simulink model "FCS"  (Simulink 9.1)
settings: Solver=VariableStepAuto  StartTime=0.0  StopTime=10.0  RelTol=1e-3
values from neighbouring files (symbols this model uses):
  Controller =     [data_set.mat]
  Estimator =     [data_set.mat]
  g = 9.81    [data_set.mat]
  init =     [data_set.mat]
  Sensors =     [data_set.mat]
  Ts = 0.005    [data_set.mat]
  Vehicle =     [data_set.mat]
undefined symbols (not defined in the file or in its folder): DiscIntNeverNeededParam, Discrete, Time
libraries: F_Line_block x503, simulink x33, ctrlSharedLib x3, sharedtransform x3, sharedutil x1
(part 2 of 3)

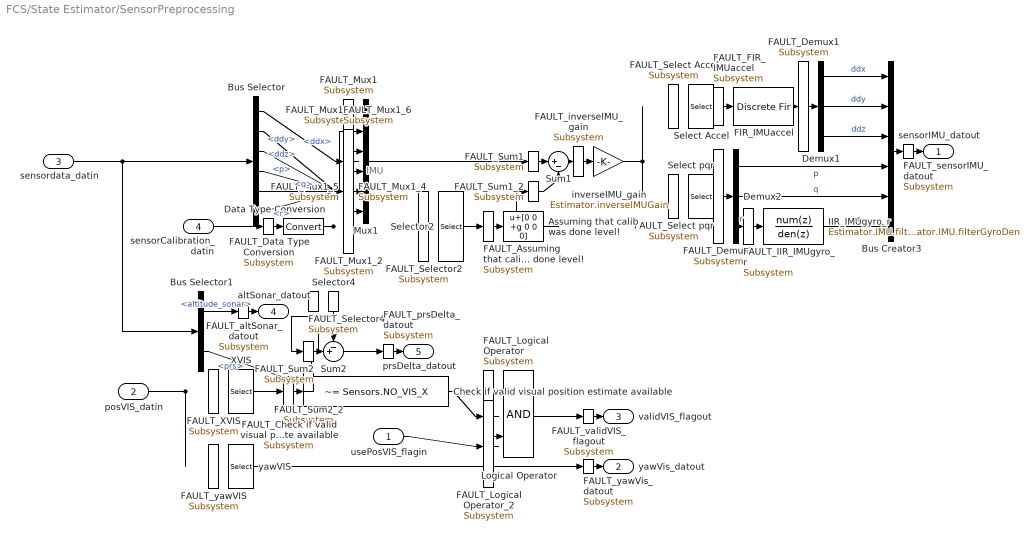
== system FCS/State Estimator/SensorPreprocessing ==
  note: IMU
  usePosVIS_flagin : Inport
  posVIS_datin : Inport  Port=2
  sensordata_datin : Inport  Port=3
  sensorCalibration_datin : Inport  Port=4
  Assuming that calib was done level! : Bias  Bias=[0 0 +g 0 0 0]
  FAULT_Assuming that calib was done level! : F_Line_block/Subsystem
  Bus Creator3 : BusCreator  Inputs=6
  Bus Selector : BusSelector  OutputSignals=ddx,ddy,ddz,p,q,r
  Bus Selector1 : BusSelector  OutputSignals=altitude_sonar,prs
  Check if valid visual position estimate available : simulink/Logic and Bit Operations/Compare To Constant  relop=~=  const=Sensors.NO_VIS_X  OutDataTypeStr=boolean
  FAULT_Check if valid visual position estimate available : F_Line_block/Subsystem
  Data Type Conversion : DataTypeConversion
  FAULT_Data Type Conversion : F_Line_block/Subsystem
  Demux1 : Demux  Outputs=3
  FAULT_Demux1 : F_Line_block/Subsystem
  Demux2 : Demux  Outputs=3
  FAULT_Demux2 : F_Line_block/Subsystem
  FIR_IMUaccel : DiscreteFir  Coefficients=Estimator.IMU.filterAccel.Coefficients
  FAULT_FIR_IMUaccel : F_Line_block/Subsystem
  IIR_IMUgyro_r : DiscreteFilter  Numerator=Estimator.IMU.filterGyroNum  Denominator=Estimator.IMU.filterGyroDen
  FAULT_IIR_IMUgyro_r : F_Line_block/Subsystem
  Logical Operator : Logic  AllPortsSameDT=off  OutDataTypeStr=boolean
  FAULT_Logical Operator : F_Line_block/Subsystem
  FAULT_Logical Operator_2 : F_Line_block/Subsystem
  Mux1 : Mux  Inputs=6
  FAULT_Mux1 : F_Line_block/Subsystem
  FAULT_Mux1_{2..6} (5 alike) : F_Line_block/Subsystem
  Select Accel : Selector  InputPortWidth=6  IndexOptions=Index vector (dialog)  Indices=[1 2 3]  OutputSizes=1
  FAULT_Select Accel : F_Line_block/Subsystem
  Select pqr : Selector  InputPortWidth=6  IndexOptions=Index vector (dialog)  Indices=[4 5 6]  OutputSizes=1
  FAULT_Select pqr : F_Line_block/Subsystem
  Selector2 : Selector  InputPortWidth=8  IndexOptions=Index vector (dialog)  Indices=[1:6]  OutputSizes=1
  FAULT_Selector2 : F_Line_block/Subsystem
  Selector4 : Selector  InputPortWidth=8  IndexOptions=Index vector (dialog)  Indices=[7]  OutputSizes=1
  FAULT_Selector4 : F_Line_block/Subsystem
  Sum1 : Sum  Inputs=|+-
  FAULT_Sum1 : F_Line_block/Subsystem
  FAULT_Sum1_2 : F_Line_block/Subsystem
  Sum2 : Sum  Inputs=-+|
  FAULT_Sum2 : F_Line_block/Subsystem
  FAULT_Sum2_2 : F_Line_block/Subsystem
  XVIS : Selector  InputPortWidth=4  IndexOptions=Index vector (dialog)  Indices=1  OutputSizes=1
  FAULT_XVIS : F_Line_block/Subsystem
  inverseIMU_gain : Gain  Gain=Estimator.inverseIMUGain  ParamDataTypeStr=single  OutDataTypeStr=single
  FAULT_inverseIMU_gain : F_Line_block/Subsystem
  yawVIS : Selector  InputPortWidth=4  IndexOptions=Index vector (dialog)  Indices=4  OutputSizes=1
  FAULT_yawVIS : F_Line_block/Subsystem
  sensorIMU_datout : Outport
  FAULT_sensorIMU_datout : F_Line_block/Subsystem
  yawVis_datout : Outport  Port=2
  FAULT_yawVis_datout : F_Line_block/Subsystem
  validVIS_flagout : Outport  Port=3
  FAULT_validVIS_flagout : F_Line_block/Subsystem
  altSonar_datout : Outport  Port=4
  FAULT_altSonar_datout : F_Line_block/Subsystem
  prsDelta_datout : Outport  Port=5
  FAULT_prsDelta_datout : F_Line_block/Subsystem
  wires:
  Select pqr/1 -> FAULT_Demux2/1
  ?FAULT_dxy_estimout_		DstPort			1/1 -> ?dxy_estimout/dstport			1
  ?FAULT_KalmanFilter_posxy/1 -> ?KalmanFilter_posxy/1
  FAULT_Demux2/1 -> Demux2/1
  Assuming that calib was done level!/1 -> FAULT_Sum1_2/1
  FAULT_Sum1_2/1 -> Sum1/2
  usePosVIS_flagin/1 -> FAULT_Logical Operator_2/1
  FAULT_Logical Operator_2/1 -> Logical Operator/2
  Check if valid visual position estimate available/1 -> FAULT_Logical Operator/1
  FAULT_Logical Operator/1 -> Logical Operator/1
  Logical Operator/1 -> FAULT_validVIS_flagout/1
  FAULT_validVIS_flagout/1 -> validVIS_flagout/1
  yawVIS/1 -> FAULT_yawVis_datout/1
  FAULT_yawVis_datout/1 -> yawVis_datout/1
  XVIS/1 -> FAULT_Check if valid visual position estimate available/1
  FAULT_Check if valid visual position estimate available/1 -> Check if valid visual position estimate available/1
  Mux1/1 -> FAULT_Sum1/1
  FAULT_Sum1/1 -> Sum1/1
  Sum2/1 -> FAULT_prsDelta_datout/1
  FAULT_prsDelta_datout/1 -> prsDelta_datout/1
  Bus Selector1/2 -> FAULT_Sum2_2/1  "<prs>"
  FAULT_Sum2_2/1 -> Sum2/2
  Selector4/1 -> FAULT_Sum2/1
  FAULT_Sum2/1 -> Sum2/1
  Bus Selector1/1 -> FAULT_altSonar_datout/1  "<altitude_sonar>"
  FAULT_altSonar_datout/1 -> altSonar_datout/1
  sensordata_datin/1 -> Bus Selector1/1, Bus Selector/1
  Bus Selector/6 -> FAULT_Mux1_6/1  "<r>"
  ?FAULT_dxy_estimout_		DstPort			1/1 -> ?dxy_estimout/dstport			1
  ?FAULT_KalmanFilter_posxy/1 -> ?KalmanFilter_posxy/1
  FAULT_Mux1_6/1 -> Mux1/6
  Bus Selector/5 -> FAULT_Mux1_5/1  "<q>"
  FAULT_Mux1_5/1 -> Mux1/5
  Bus Selector/4 -> FAULT_Mux1_4/1  "<p>"
  FAULT_Mux1_4/1 -> Mux1/4
  Bus Selector/3 -> FAULT_Mux1_3/1  "<ddz>"
  FAULT_Mux1_3/1 -> Mux1/3
  Bus Selector/2 -> FAULT_Mux1_2/1  "<ddy>"
  FAULT_Mux1_2/1 -> Mux1/2
  Bus Selector/1 -> FAULT_Mux1/1  "<ddx>"
  FAULT_Mux1/1 -> Mux1/1
  sensorCalibration_datin/1 -> FAULT_Data Type Conversion/1
  FAULT_Data Type Conversion/1 -> Data Type Conversion/1
  IIR_IMUgyro_r/1 -> Bus Creator3/6  "r"
  Demux2/3 -> FAULT_IIR_IMUgyro_r/1  "r"
  FAULT_IIR_IMUgyro_r/1 -> IIR_IMUgyro_r/1
  FIR_IMUaccel/1 -> FAULT_Demux1/1
  FAULT_Demux1/1 -> Demux1/1
  Select Accel/1 -> FAULT_FIR_IMUaccel/1
  FAULT_FIR_IMUaccel/1 -> FIR_IMUaccel/1
  inverseIMU_gain/1 -> ?FAULT_Select Accel_		DstPort			1/1, ?FAULT_Select pqr_		DstPort			1/1
  ?FAULT_Select Accel_		DstPort			1/1 -> Select Accel/dstport			1
  ?FAULT_Select pqr_		DstPort			1/1 -> Select pqr/dstport			1
  Demux2/2 -> Bus Creator3/5  "q"
  Demux2/1 -> Bus Creator3/4  "p"
  Selector2/1 -> FAULT_Assuming that calib was done level!/1
  FAULT_Assuming that calib was done level!/1 -> Assuming that calib was done level!/1
  Sum1/1 -> FAULT_inverseIMU_gain/1
  FAULT_inverseIMU_gain/1 -> inverseIMU_gain/1
  Demux1/3 -> Bus Creator3/3  "ddz"
  Demux1/2 -> Bus Creator3/2  "ddy"
  Demux1/1 -> Bus Creator3/1  "ddx"
  Bus Creator3/1 -> FAULT_sensorIMU_datout/1
  FAULT_sensorIMU_datout/1 -> sensorIMU_datout/1
  posVIS_datin/1 -> ?FAULT_XVIS_		DstPort			1/1, ?FAULT_yawVIS_		DstPort			1/1
  ?FAULT_XVIS_		DstPort			1/1 -> XVIS/dstport			1
  ?FAULT_yawVIS_		DstPort			1/1 -> yawVIS/dstport			1
  Data Type Conversion/1 -> ?FAULT_Selector2_		DstPort			1/1, ?FAULT_Selector4_		DstPort			1/1
  ?FAULT_Selector2_		DstPort			1/1 -> Selector2/dstport			1
  ?FAULT_Selector4_		DstPort			1/1 -> Selector4/dstport			1

== system FCS/controller/Attitude ==
  note: ATTITUDE
  refAttitude : Inport
  states_estim : Inport  Port=2
  Add : Sum  Inputs=+-
  FAULT_Add : F_Line_block/Subsystem
  FAULT_Add_2 : F_Line_block/Subsystem
  Bus Selector3 : BusSelector  OutputSignals=pitch,roll
  Bus Selector4 : BusSelector  OutputSignals=q,p
  D_pr : Gain  Gain=[0.002;0.003]
  FAULT_D_pr : F_Line_block/Subsystem
  Delay : Delay  DelayLength=1  InitialCondition=0
  FAULT_Delay : F_Line_block/Subsystem
  Demux : Demux  Outputs=2
  FAULT_Demux : F_Line_block/Subsystem
  Discrete-Time Integrator : DiscreteIntegrator  SampleTime=Ts  LimitOutput=on  UpperSaturationLimit=2  LowerSaturationLimit=-2  ICPrevOutput=DiscIntNeverNeededParam  ICPrevScaledInput=DiscIntNeverNeededParam
  FAULT_Discrete-Time Integrator : F_Line_block/Subsystem
  I_pr : Gain  Gain=0.01
  FAULT_I_pr : F_Line_block/Subsystem
  Mux : Mux  Inputs=2
  FAULT_Mux : F_Line_block/Subsystem
  FAULT_Mux_2 : F_Line_block/Subsystem
  Mux1 : Mux  Inputs=2
  FAULT_Mux1 : F_Line_block/Subsystem
  FAULT_Mux1_2 : F_Line_block/Subsystem
  P_pr : Gain  Gain=[0.013;0.02]
  FAULT_P_pr : F_Line_block/Subsystem
  Sum16 : Sum  Inputs=++-  AccumDataTypeStr=single  OutDataTypeStr=single  SaturateOnIntegerOverflow=on
  FAULT_Sum16 : F_Line_block/Subsystem
  FAULT_Sum16_2 : F_Line_block/Subsystem
  FAULT_Sum16_3 : F_Line_block/Subsystem
  Sum19 : Sum  Inputs=+-|
  FAULT_Sum19 : F_Line_block/Subsystem
  FAULT_Sum19_2 : F_Line_block/Subsystem
  antiWU_Gain : Gain  Gain=0.001
  FAULT_antiWU_Gain : F_Line_block/Subsystem
  tau_pitch : Outport
  FAULT_tau_pitch : F_Line_block/Subsystem
  tau_roll : Outport  Port=2
  FAULT_tau_roll : F_Line_block/Subsystem
  wires:
  Sum16/1 -> FAULT_Demux/1  "P_pr"
  FAULT_Demux/1 -> Demux/1
  antiWU_Gain/1 -> FAULT_Add_2/1
  FAULT_Add_2/1 -> Add/2
  Add/1 -> FAULT_Discrete-Time Integrator/1
  FAULT_Discrete-Time Integrator/1 -> Discrete-Time Integrator/1
  Bus Selector3/1 -> FAULT_Mux/1  "<pitch>"
  FAULT_Mux/1 -> Mux/1
  Bus Selector4/1 -> FAULT_Mux1/1  "<q>"
  FAULT_Mux1/1 -> Mux1/1
  P_pr/1 -> FAULT_Sum16/1
  FAULT_Sum16/1 -> Sum16/1
  I_pr/1 -> FAULT_Sum16_2/1
  FAULT_Sum16_2/1 -> Sum16/2
  Sum19/1 -> ?FAULT_Add_		DstPort			1/1, ?FAULT_P_pr_		DstPort			1/1  "pitch/roll error"
  ?FAULT_Add_		DstPort			1/1 -> Add/dstport			1
  ?FAULT_P_pr_		DstPort			1/1 -> P_pr/dstport			1
  Discrete-Time Integrator/1 -> ?FAULT_Delay_		DstPort			1/1, ?FAULT_I_pr_		DstPort			1/1
  ?FAULT_Delay_		DstPort			1/1 -> Delay/dstport			1
  ?FAULT_I_pr_		DstPort			1/1 -> I_pr/dstport			1
  Delay/1 -> FAULT_antiWU_Gain/1
  FAULT_antiWU_Gain/1 -> antiWU_Gain/1
  Demux/1 -> FAULT_tau_pitch/1  "tau_pitch"
  FAULT_tau_pitch/1 -> tau_pitch/1
  Demux/2 -> FAULT_tau_roll/1
  FAULT_tau_roll/1 -> tau_roll/1
  D_pr/1 -> FAULT_Sum16_3/1
  FAULT_Sum16_3/1 -> Sum16/3
  states_estim/1 -> Bus Selector3/1, Bus Selector4/1
  refAttitude/1 -> FAULT_Sum19/1
  ?FAULT_Delay_		DstPort			1/1 -> Delay/dstport			1
  ?FAULT_I_pr_		DstPort			1/1 -> I_pr/dstport			1
  FAULT_Sum19/1 -> Sum19/1
  Mux/1 -> FAULT_Sum19_2/1
  FAULT_Sum19_2/1 -> Sum19/2
  Bus Selector3/2 -> FAULT_Mux_2/1  "<roll>"
  FAULT_Mux_2/1 -> Mux/2
  Mux1/1 -> FAULT_D_pr/1
  FAULT_D_pr/1 -> D_pr/1
  Bus Selector4/2 -> FAULT_Mux1_2/1  "<p>"
  FAULT_Mux1_2/1 -> Mux1/2

== system FCS/controller/ControlMixer ==
  tau_pitch : Inport
  tau_roll : Inport  Port=2
  tau_yaw : Inport  Port=3
  totalThrust : Inport  Port=4
  Mux2 : Mux
  FAULT_Mux2 : F_Line_block/Subsystem
  FAULT_Mux2_2 : F_Line_block/Subsystem
  FAULT_Mux2_3 : F_Line_block/Subsystem
  FAULT_Mux2_4 : F_Line_block/Subsystem
  Product : Product  Multiplication=Matrix(*)  RndMeth=Zero
  FAULT_Product : F_Line_block/Subsystem
  FAULT_Product_2 : F_Line_block/Subsystem
  TorqueTotalThrustToThrustPerMotor : Constant  Value=Controller.Q2Ts  OutDataTypeStr=single
  thrusts_refout : Outport
  FAULT_thrusts_refout : F_Line_block/Subsystem
  wires:
  Product/1 -> FAULT_thrusts_refout/1
  FAULT_thrusts_refout/1 -> thrusts_refout/1
  tau_roll/1 -> FAULT_Mux2_4/1
  FAULT_Mux2_4/1 -> Mux2/4
  tau_pitch/1 -> FAULT_Mux2_3/1
  FAULT_Mux2_3/1 -> Mux2/3
  tau_yaw/1 -> FAULT_Mux2_2/1
  FAULT_Mux2_2/1 -> Mux2/2
  totalThrust/1 -> FAULT_Mux2/1
  FAULT_Mux2/1 -> Mux2/1
  TorqueTotalThrustToThrustPerMotor/1 -> FAULT_Product/1
  FAULT_Product/1 -> Product/1
  Mux2/1 -> FAULT_Product_2/1
  FAULT_Product_2/1 -> Product/2

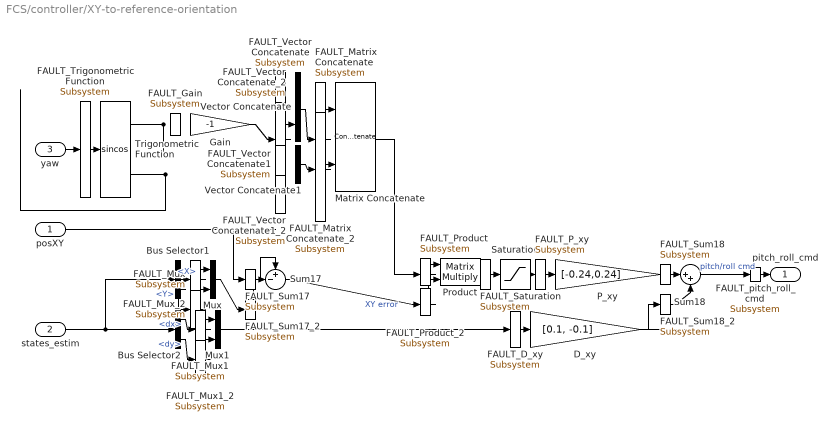
== system FCS/controller/XY-to-reference-orientation ==
  posXY : Inport
  states_estim : Inport  Port=2
  yaw : Inport  Port=3
  Bus Selector1 : BusSelector  OutputSignals=X,Y
  Bus Selector2 : BusSelector  OutputSignals=dx,dy
  D_xy : Gain  Gain=[0.1, -0.1]  ParamDataTypeStr=single  OutDataTypeStr=single  SaturateOnIntegerOverflow=on
  FAULT_D_xy : F_Line_block/Subsystem
  Gain : Gain  Gain=-1
  FAULT_Gain : F_Line_block/Subsystem
  Matrix Concatenate : Concatenate  Mode=Multidimensional array  ConcatenateDimension=2
  FAULT_Matrix Concatenate : F_Line_block/Subsystem
  FAULT_Matrix Concatenate_2 : F_Line_block/Subsystem
  Mux : Mux  Inputs=2
  FAULT_Mux : F_Line_block/Subsystem
  FAULT_Mux_2 : F_Line_block/Subsystem
  Mux1 : Mux  Inputs=2
  FAULT_Mux1 : F_Line_block/Subsystem
  FAULT_Mux1_2 : F_Line_block/Subsystem
  P_xy : Gain  Gain=[-0.24,0.24]  ParamDataTypeStr=single  OutDataTypeStr=single  SaturateOnIntegerOverflow=on
  FAULT_P_xy : F_Line_block/Subsystem
  Product : Product  Multiplication=Matrix(*)  OutDataTypeStr=single  RndMeth=Zero
  FAULT_Product : F_Line_block/Subsystem
  FAULT_Product_2 : F_Line_block/Subsystem
  Saturation : Saturate  UpperLimit=3  LowerLimit=-3  OutDataTypeStr=single
  FAULT_Saturation : F_Line_block/Subsystem
  Sum17 : Sum  Inputs=+-|  AccumDataTypeStr=single
  FAULT_Sum17 : F_Line_block/Subsystem
  FAULT_Sum17_2 : F_Line_block/Subsystem
  Sum18 : Sum  Inputs=|++  AccumDataTypeStr=single  OutDataTypeStr=single  SaturateOnIntegerOverflow=on
  FAULT_Sum18 : F_Line_block/Subsystem
  FAULT_Sum18_2 : F_Line_block/Subsystem
  Trigonometric Function : Trigonometry  Operator=sincos
  FAULT_Trigonometric Function : F_Line_block/Subsystem
  Vector Concatenate : Concatenate
  FAULT_Vector Concatenate : F_Line_block/Subsystem
  FAULT_Vector Concatenate_2 : F_Line_block/Subsystem
  Vector Concatenate1 : Concatenate
  FAULT_Vector Concatenate1 : F_Line_block/Subsystem
  FAULT_Vector Concatenate1_2 : F_Line_block/Subsystem
  pitch_roll_cmd : Outport
  FAULT_pitch_roll_cmd : F_Line_block/Subsystem
  wires:
  yaw/1 -> FAULT_Trigonometric Function/1
  FAULT_Trigonometric Function/1 -> Trigonometric Function/1
  Saturation/1 -> FAULT_P_xy/1
  FAULT_P_xy/1 -> P_xy/1
  P_xy/1 -> FAULT_Sum18/1
  FAULT_Sum18/1 -> Sum18/1
  Sum17/1 -> FAULT_Product_2/1  "XY error"
  FAULT_Product_2/1 -> Product/2
  posXY/1 -> FAULT_Sum17/1
  FAULT_Sum17/1 -> Sum17/1
  Bus Selector2/1 -> FAULT_Mux1/1  "<dx>"
  FAULT_Mux1/1 -> Mux1/1
  states_estim/1 -> Bus Selector1/1, Bus Selector2/1
  Sum18/1 -> FAULT_pitch_roll_cmd/1  "pitch/roll cmd"
  ?FAULT_Delay_		DstPort			1/1 -> ?Delay/dstport			1
  ?FAULT_I_pr_		DstPort			1/1 -> ?I_pr/dstport			1
  FAULT_pitch_roll_cmd/1 -> pitch_roll_cmd/1
  D_xy/1 -> FAULT_Sum18_2/1
  FAULT_Sum18_2/1 -> Sum18/2
  Bus Selector1/1 -> FAULT_Mux/1  "<X>"
  FAULT_Mux/1 -> Mux/1
  Product/1 -> FAULT_Saturation/1
  FAULT_Saturation/1 -> Saturation/1
  Trigonometric Function/1 -> ?FAULT_Gain_		DstPort			1/1, ?FAULT_Vector Concatenate1_		DstPort			1/1
  ?FAULT_Gain_		DstPort			1/1 -> Gain/dstport			1
  ?FAULT_Vector Concatenate1_		DstPort			1/1 -> Vector Concatenate1/dstport			1
  Trigonometric Function/2 -> ?FAULT_Vector Concatenate1_		DstPort			2/1, ?FAULT_Vector Concatenate_		DstPort			1/1
  ?FAULT_Vector Concatenate1_		DstPort			2/1 -> Vector Concatenate1/dstport			2
  ?FAULT_Vector Concatenate_		DstPort			1/1 -> Vector Concatenate/dstport			1
  Gain/1 -> FAULT_Vector Concatenate_2/1
  FAULT_Vector Concatenate_2/1 -> Vector Concatenate/2
  Vector Concatenate/1 -> FAULT_Matrix Concatenate/1
  FAULT_Matrix Concatenate/1 -> Matrix Concatenate/1
  Vector Concatenate1/1 -> FAULT_Matrix Concatenate_2/1
  FAULT_Matrix Concatenate_2/1 -> Matrix Concatenate/2
  Matrix Concatenate/1 -> FAULT_Product/1
  FAULT_Product/1 -> Product/1
  Bus Selector1/2 -> FAULT_Mux_2/1  "<Y>"
  FAULT_Mux_2/1 -> Mux/2
  Mux/1 -> FAULT_Sum17_2/1
  FAULT_Sum17_2/1 -> Sum17/2
  Mux1/1 -> FAULT_D_xy/1
  FAULT_D_xy/1 -> D_xy/1
  Bus Selector2/2 -> FAULT_Mux1_2/1  "<dy>"
  FAULT_Mux1_2/1 -> Mux1/2

== system FCS/controller/Yaw ==
  yaw_ref : Inport
  states_estim : Inport  Port=2
  Bus Selector5 : BusSelector  OutputSignals=yaw,r
  D_yaw : Gain  Gain=0.3*0.004
  FAULT_D_yaw : F_Line_block/Subsystem
  P_yaw : Gain  Gain=0.004  ParamDataTypeStr=single  OutDataTypeStr=single
  FAULT_P_yaw : F_Line_block/Subsystem
  Sum1 : Sum  Inputs=+-|  AccumDataTypeStr=single  OutDataTypeStr=single  SaturateOnIntegerOverflow=on
  FAULT_Sum1 : F_Line_block/Subsystem
  FAULT_Sum1_2 : F_Line_block/Subsystem
  Sum2 : Sum  Inputs=|+-
  FAULT_Sum2 : F_Line_block/Subsystem
  FAULT_Sum2_2 : F_Line_block/Subsystem
  yaw : Outport
  FAULT_yaw : F_Line_block/Subsystem
  tau_yaw : Outport  Port=2
  FAULT_tau_yaw : F_Line_block/Subsystem
  wires:
  D_yaw/1 -> FAULT_Sum2_2/1
  FAULT_Sum2_2/1 -> Sum2/2
  P_yaw/1 -> FAULT_Sum2/1
  FAULT_Sum2/1 -> Sum2/1
  Bus Selector5/2 -> FAULT_D_yaw/1  "<r>"
  FAULT_D_yaw/1 -> D_yaw/1
  Sum1/1 -> FAULT_P_yaw/1
  FAULT_P_yaw/1 -> P_yaw/1
  states_estim/1 -> Bus Selector5/1
  Sum2/1 -> FAULT_tau_yaw/1
  FAULT_tau_yaw/1 -> tau_yaw/1
  Bus Selector5/1 -> ?FAULT_yaw_		DstPort			1/1, ?FAULT_Sum1_		DstPort			2/1  "<yaw>"
  ?FAULT_yaw_		DstPort			1/1 -> yaw/dstport			1
  ?FAULT_Sum1_		DstPort			2/1 -> Sum1/dstport			2
  yaw_ref/1 -> FAULT_Sum1/1
  FAULT_Sum1/1 -> Sum1/1

== system FCS/controller/gravity feedforward/equilibrium thrust ==
  note: ALTITUDE
  states_estim : Inport
  PosZ : Inport  Port=2
  takeoff_flag : Inport  Port=3
  Bus Selector6 : BusSelector  OutputSignals=Z,dz
  D_z : Gain  Gain=0.3  ParamDataTypeStr=single  OutDataTypeStr=single  SaturateOnIntegerOverflow=on
  FAULT_D_z : F_Line_block/Subsystem
  P_z : Gain  Gain=0.8  ParamDataTypeStr=single  OutDataTypeStr=single  SaturateOnIntegerOverflow=on
  FAULT_P_z : F_Line_block/Subsystem
  SaturationThrust : Saturate  UpperLimit=4*Controller.totalThrustMaxRelative*Controller.motorsThrustPerMotorMax  LowerLimit=-4*Controller.totalThrustMaxRelative*Controller.motorsThrustPerMotorMax  OutDataTypeStr=single
  FAULT_SaturationThrust : F_Line_block/Subsystem
  Sum15 : Sum  Inputs=|+-  AccumDataTypeStr=single  OutDataTypeStr=single  SaturateOnIntegerOverflow=on
  FAULT_Sum15 : F_Line_block/Subsystem
  FAULT_Sum15_2 : F_Line_block/Subsystem
  Sum3 : Sum  Inputs=+-|  AccumDataTypeStr=single  OutDataTypeStr=single  SaturateOnIntegerOverflow=on
  FAULT_Sum3 : F_Line_block/Subsystem
  FAULT_Sum3_2 : F_Line_block/Subsystem
  Sum4 : Sum  Inputs=++|  AccumDataTypeStr=single  OutDataTypeStr=single  SaturateOnIntegerOverflow=on
  FAULT_Sum4 : F_Line_block/Subsystem
  FAULT_Sum4_2 : F_Line_block/Subsystem
  TakeoffOrControl_Switch : Switch  Criteria=u2 > Threshold
  takeoff_gain : Gain  Gain=Controller.takeoffGain  ParamDataTypeStr=single  OutDataTypeStr=single  SaturateOnIntegerOverflow=on
  FAULT_takeoff_gain : F_Line_block/Subsystem
  w0 : Constant  Value=-g*Vehicle.Airframe.mass  OutDataTypeStr=single  SampleTime=Ts
  altitude_cmd : Outport
  FAULT_altitude_cmd : F_Line_block/Subsystem
  wires:
  Sum3/1 -> FAULT_P_z/1  "errZ"
  FAULT_P_z/1 -> P_z/1
  TakeoffOrControl_Switch/1 -> FAULT_Sum4_2/1
  FAULT_Sum4_2/1 -> Sum4/2
  Bus Selector6/1 -> FAULT_Sum3_2/1  "<Z>"
  FAULT_Sum3_2/1 -> Sum3/2
  Bus Selector6/2 -> FAULT_D_z/1  "<dz>"
  FAULT_D_z/1 -> D_z/1
  w0/1 -> ?FAULT_Sum4_		DstPort			1/1, ?FAULT_takeoff_gain_		DstPort			1/1
  ?FAULT_Sum4_		DstPort			1/1 -> Sum4/dstport			1
  ?FAULT_takeoff_gain_		DstPort			1/1 -> takeoff_gain/dstport			1
  D_z/1 -> FAULT_Sum15_2/1  "dz"
  FAULT_Sum15_2/1 -> Sum15/2
  takeoff_gain/1 -> TakeoffOrControl_Switch/1
  takeoff_flag/1 -> TakeoffOrControl_Switch/2
  PosZ/1 -> FAULT_Sum3/1
  FAULT_Sum3/1 -> Sum3/1
  P_z/1 -> FAULT_Sum15/1
  FAULT_Sum15/1 -> Sum15/1
  Sum15/1 -> TakeoffOrControl_Switch/3
  Sum4/1 -> FAULT_SaturationThrust/1
  FAULT_SaturationThrust/1 -> SaturationThrust/1
  SaturationThrust/1 -> FAULT_altitude_cmd/1
  FAULT_altitude_cmd/1 -> altitude_cmd/1
  states_estim/1 -> Bus Selector6/1

== system FCS/controller/thrustsToMotorCommands ==
  thrusts_refin : Inport
  MotorDirections : Gain  Gain=[1 -1 1 -1]
  FAULT_MotorDirections : F_Line_block/Subsystem
  Saturation5 : Saturate  UpperLimit=Vehicle.Motor.maxLimit  LowerLimit=Vehicle.Motor.minLimit
  FAULT_Saturation5 : F_Line_block/Subsystem
  ThrustToMotorCommand : Gain  Gain=-Vehicle.Motor.thrustToMotorCommand
  FAULT_ThrustToMotorCommand : F_Line_block/Subsystem
  motors_cmdout : Outport
  FAULT_motors_cmdout : F_Line_block/Subsystem
  wires:
  Saturation5/1 -> FAULT_MotorDirections/1
  FAULT_MotorDirections/1 -> MotorDirections/1
  MotorDirections/1 -> FAULT_motors_cmdout/1
  FAULT_motors_cmdout/1 -> motors_cmdout/1
  ThrustToMotorCommand/1 -> FAULT_Saturation5/1
  FAULT_Saturation5/1 -> Saturation5/1
  thrusts_refin/1 -> FAULT_ThrustToMotorCommand/1
  FAULT_ThrustToMotorCommand/1 -> ThrustToMotorCommand/1

== system FCS/State Estimator/Complementary Filter/If Action Subsystem ==
  rpy : Inport
  accel : Inport  Port=2
  Action Port : ActionPort
  FAULT_Action Port : F_Line_block/Subsystem
  Demux : Demux  Outputs=3
  FAULT_Demux : F_Line_block/Subsystem
  Demux1 : Demux  Outputs=3
  FAULT_Demux1 : F_Line_block/Subsystem
  Divide : Product  Inputs=*/
  FAULT_Divide : F_Line_block/Subsystem
  FAULT_Divide_2 : F_Line_block/Subsystem
  Gain : Gain  Gain=1-Estimator.gyroAngleUpdateAccWeight
  FAULT_Gain{,1..4} (5 alike) : F_Line_block/Subsystem
  Gain1 : Gain  Gain=Estimator.gyroAngleUpdateAccWeight
  Gain2 : Gain  Gain=1/g
  Gain3 : Gain  Gain=Estimator.gyroAngleUpdateAccWeight
  Gain4 : Gain  Gain=1-Estimator.gyroAngleUpdateAccWeight
  Mux : Mux  Inputs=2
  FAULT_Mux : F_Line_block/Subsystem
  FAULT_Mux_2 : F_Line_block/Subsystem
  Sum : Sum  Inputs=|++
  FAULT_Sum : F_Line_block/Subsystem
  FAULT_Sum_2 : F_Line_block/Subsystem
  Sum1 : Sum  Inputs=|++
  FAULT_Sum1 : F_Line_block/Subsystem
  FAULT_Sum1_2 : F_Line_block/Subsystem
  Terminator1 : Terminator
  FAULT_Terminator1 : F_Line_block/Subsystem
  Trigonometric Function : Trigonometry  Operator=atan
  FAULT_Trigonometric Function : F_Line_block/Subsystem
  Trigonometric Function1 : Trigonometry  Operator=asin
  FAULT_Trigonometric Function1 : F_Line_block/Subsystem
  pitch,roll : Outport
  FAULT_pitch,roll : F_Line_block/Subsystem
  wires:
  accel/1 -> FAULT_Demux/1
  FAULT_Demux/1 -> Demux/1
  Demux/2 -> FAULT_Divide/1
  FAULT_Divide/1 -> Divide/1
  Demux/3 -> FAULT_Divide_2/1
  FAULT_Divide_2/1 -> Divide/2
  Divide/1 -> FAULT_Trigonometric Function/1
  FAULT_Trigonometric Function/1 -> Trigonometric Function/1
  Gain/1 -> FAULT_Sum/1
  FAULT_Sum/1 -> Sum/1
  Trigonometric Function/1 -> FAULT_Gain1/1
  FAULT_Gain1/1 -> Gain1/1
  Mux/1 -> FAULT_pitch,roll/1
  FAULT_pitch,roll/1 -> pitch,roll/1
  Gain2/1 -> FAULT_Trigonometric Function1/1
  FAULT_Trigonometric Function1/1 -> Trigonometric Function1/1
  Trigonometric Function1/1 -> FAULT_Gain3/1
  FAULT_Gain3/1 -> Gain3/1
  Gain4/1 -> FAULT_Sum1/1
  FAULT_Sum1/1 -> Sum1/1
  Gain3/1 -> FAULT_Sum1_2/1
  FAULT_Sum1_2/1 -> Sum1/2
  Sum1/1 -> FAULT_Mux/1
  FAULT_Mux/1 -> Mux/1
  Sum/1 -> FAULT_Mux_2/1
  FAULT_Mux_2/1 -> Mux/2
  rpy/1 -> FAULT_Demux1/1
  FAULT_Demux1/1 -> Demux1/1
  Demux1/1 -> FAULT_Gain/1
  FAULT_Gain/1 -> Gain/1
  Demux1/2 -> FAULT_Gain4/1
  FAULT_Gain4/1 -> Gain4/1
  Demux/1 -> FAULT_Gain2/1
  FAULT_Gain2/1 -> Gain2/1
  Demux1/3 -> FAULT_Terminator1/1
  FAULT_Terminator1/1 -> Terminator1/1
  Gain1/1 -> FAULT_Sum_2/1
  FAULT_Sum_2/1 -> Sum/2

== system FCS/State Estimator/Complementary Filter/If Action Subsystem1 ==
  rpy : Inport
  yawVis : Inport  Port=2
  Action Port : ActionPort
  FAULT_Action Port : F_Line_block/Subsystem
  Gain : Gain  Gain=1-Estimator.gyroAngleUpdateVisWeight
  FAULT_Gain : F_Line_block/Subsystem
  Gain1 : Gain  Gain=Estimator.gyroAngleUpdateVisWeight
  FAULT_Gain1 : F_Line_block/Subsystem
  Selector4 : Selector  InputPortWidth=3  IndexOptions=Index vector (dialog)  Indices=[3]  OutputSizes=1
  FAULT_Selector4 : F_Line_block/Subsystem
  Sum : Sum  Inputs=|++
  FAULT_Sum : F_Line_block/Subsystem
  FAULT_Sum_2 : F_Line_block/Subsystem
  yaw : Outport
  FAULT_yaw : F_Line_block/Subsystem
  wires:
  rpy/1 -> FAULT_Selector4/1
  FAULT_Selector4/1 -> Selector4/1
  Selector4/1 -> FAULT_Gain/1
  FAULT_Gain/1 -> Gain/1
  yawVis/1 -> FAULT_Gain1/1
  FAULT_Gain1/1 -> Gain1/1
  Gain/1 -> FAULT_Sum/1
  FAULT_Sum/1 -> Sum/1
  Gain1/1 -> FAULT_Sum_2/1
  FAULT_Sum_2/1 -> Sum/2
  Sum/1 -> FAULT_yaw/1
  FAULT_yaw/1 -> yaw/1

== system FCS/State Estimator/Complementary Filter/If Action Subsystem2 ==
  prin : Inport
  Action Port : ActionPort
  FAULT_Action Port : F_Line_block/Subsystem
  prout : Outport
  FAULT_prout : F_Line_block/Subsystem
  wires:
  prin/1 -> FAULT_prout/1
  FAULT_prout/1 -> prout/1

== system FCS/State Estimator/Complementary Filter/If Action Subsystem3 ==
  yawin : Inport
  Action Port : ActionPort
  FAULT_Action Port : F_Line_block/Subsystem
  yout : Outport
  FAULT_yout : F_Line_block/Subsystem
  wires:
  yawin/1 -> FAULT_yout/1
  FAULT_yout/1 -> yout/1

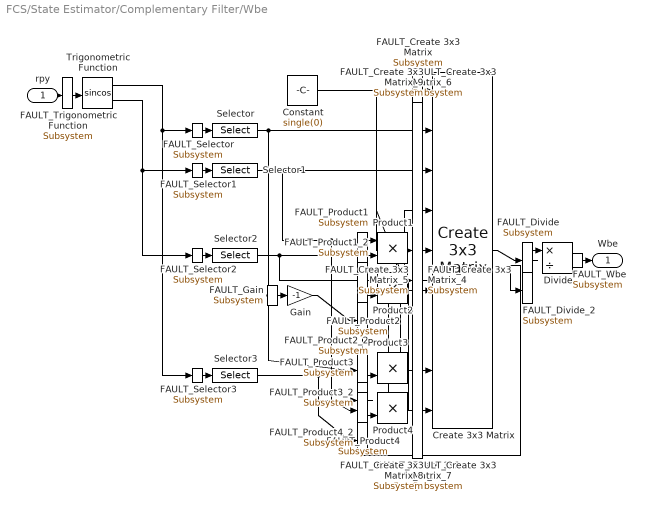
== system FCS/State Estimator/Complementary Filter/Wbe ==
  rpy : Inport  OutDataTypeStr=single
  Constant : Constant  Value=single(0)
  Create 3x3 Matrix : sharedutil/Create 3x3 Matrix  aMode=aMode
  FAULT_Create 3x3 Matrix : F_Line_block/Subsystem
  FAULT_Create 3x3 Matrix_{2..9} (8 alike) : F_Line_block/Subsystem
  Divide : Product  Inputs=*/
  FAULT_Divide : F_Line_block/Subsystem
  FAULT_Divide_2 : F_Line_block/Subsystem
  Gain : Gain  Gain=-1
  FAULT_Gain : F_Line_block/Subsystem
  Product{1..4} (4 alike) : Product
  FAULT_Product{1..4} (4 alike) : F_Line_block/Subsystem
  FAULT_Product1_2 : F_Line_block/Subsystem
  FAULT_Product2_2 : F_Line_block/Subsystem
  FAULT_Product3_2 : F_Line_block/Subsystem
  FAULT_Product4_2 : F_Line_block/Subsystem
  Selector : Selector  InputPortWidth=3  IndexOptions=Index vector (dialog)  Indices=[1]  OutputSizes=1
  FAULT_Selector{,1..3} (4 alike) : F_Line_block/Subsystem
  Selector1 : Selector  InputPortWidth=3  IndexOptions=Index vector (dialog)  Indices=[1]  OutputSizes=1
  Selector2 : Selector  InputPortWidth=3  IndexOptions=Index vector (dialog)  Indices=[2]  OutputSizes=1
  Selector3 : Selector  InputPortWidth=3  IndexOptions=Index vector (dialog)  Indices=[2]  OutputSizes=1
  Trigonometric Function : Trigonometry  Operator=sincos
  FAULT_Trigonometric Function : F_Line_block/Subsystem
  Wbe : Outport
  FAULT_Wbe : F_Line_block/Subsystem
  wires:
  Create 3x3 Matrix/1 -> FAULT_Divide/1
  FAULT_Divide/1 -> Divide/1
  Product3/1 -> FAULT_Create 3x3 Matrix_8/1
  FAULT_Create 3x3 Matrix_8/1 -> Create 3x3 Matrix/8
  Trigonometric Function/2 -> FAULT_Selector1/1, FAULT_Selector2/1
  FAULT_Selector1/1 -> Selector1/1
  FAULT_Selector2/1 -> Selector2/1
  Selector3/1 -> FAULT_Product4_2/1, FAULT_Product3_2/1
  FAULT_Product4_2/1 -> Product4/2
  FAULT_Product3_2/1 -> Product3/2
  Selector1/1 -> FAULT_Product4/1, Product1/1, Create 3x3 Matrix/3
  Trigonometric Function/1 -> FAULT_Selector3/1, FAULT_Selector/1
  FAULT_Selector3/1 -> Selector3/1
  FAULT_Selector/1 -> Selector/1
  Product1/1 -> FAULT_Create 3x3 Matrix_5/1
  FAULT_Create 3x3 Matrix_5/1 -> Create 3x3 Matrix/5
  Product2/1 -> FAULT_Create 3x3 Matrix_6/1
  FAULT_Create 3x3 Matrix_6/1 -> Create 3x3 Matrix/6
  Selector2/1 -> FAULT_Divide_2/1, FAULT_Create 3x3 Matrix_7/1, Product2/1, Product1/2
  Gain/1 -> FAULT_Product2_2/1
  FAULT_Product2_2/1 -> Product2/2
  Product4/1 -> FAULT_Create 3x3 Matrix_9/1
  FAULT_Create 3x3 Matrix_9/1 -> Create 3x3 Matrix/9
  Constant/1 -> FAULT_Create 3x3 Matrix_4/1, FAULT_Create 3x3 Matrix/1
  FAULT_Create 3x3 Matrix_4/1 -> Create 3x3 Matrix/4
  FAULT_Create 3x3 Matrix/1 -> Create 3x3 Matrix/1
  Divide/1 -> FAULT_Wbe/1
  FAULT_Wbe/1 -> Wbe/1
  rpy/1 -> FAULT_Trigonometric Function/1
  FAULT_Trigonometric Function/1 -> Trigonometric Function/1
  Selector/1 -> FAULT_Product3/1, Gain/1, Create 3x3 Matrix/2

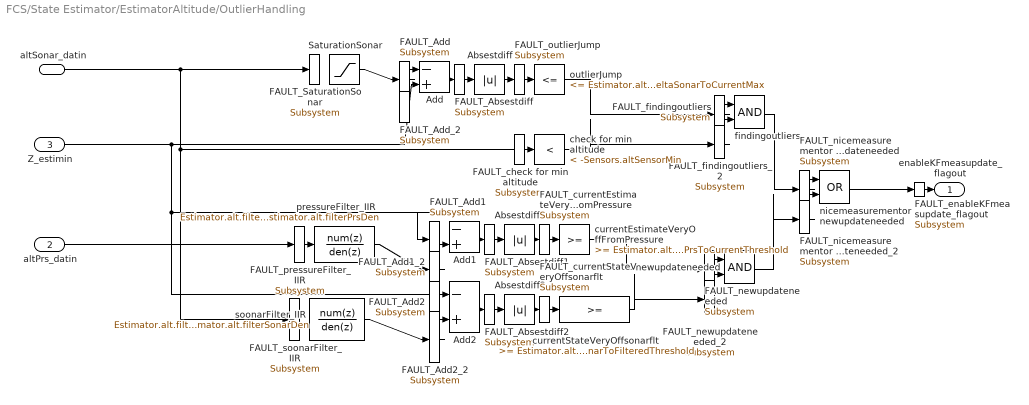
== system FCS/State Estimator/EstimatorAltitude/OutlierHandling ==
  altSonar_datin : Inport
  altPrs_datin : Inport  Port=2
  Z_estimin : Inport  Port=3
  Absestdiff : Abs
  FAULT_Absestdiff : F_Line_block/Subsystem
  Absestdiff1 : Abs
  FAULT_Absestdiff1 : F_Line_block/Subsystem
  Absestdiff2 : Abs
  FAULT_Absestdiff2 : F_Line_block/Subsystem
  Add : Sum  Inputs=-+
  FAULT_Add : F_Line_block/Subsystem
  FAULT_Add_2 : F_Line_block/Subsystem
  Add1 : Sum  Inputs=-+
  FAULT_Add1 : F_Line_block/Subsystem
  FAULT_Add1_2 : F_Line_block/Subsystem
  Add2 : Sum  Inputs=-+
  FAULT_Add2 : F_Line_block/Subsystem
  FAULT_Add2_2 : F_Line_block/Subsystem
  SaturationSonar : Saturate  UpperLimit=-Sensors.altSensorMin  LowerLimit=-inf
  FAULT_SaturationSonar : F_Line_block/Subsystem
  check for min altitude : simulink/Logic and Bit Operations/Compare To Constant  relop=<  const=-Sensors.altSensorMin  OutDataTypeStr=boolean
  FAULT_check for min altitude : F_Line_block/Subsystem
  currentEstimateVeryOffFromPressure : simulink/Logic and Bit Operations/Compare To Constant  relop=>=  const=Estimator.alt.deltaPrsToCurrentThreshold  OutDataTypeStr=boolean
  FAULT_currentEstimateVeryOffFromPressure : F_Line_block/Subsystem
  currentStateVeryOffsonarflt : simulink/Logic and Bit Operations/Compare To Constant  relop=>=  const=Estimator.alt.deltaSonarToFilteredThreshold  OutDataTypeStr=boolean
  FAULT_currentStateVeryOffsonarflt : F_Line_block/Subsystem
  findingoutliers : Logic  AllPortsSameDT=off  OutDataTypeStr=boolean
  FAULT_findingoutliers : F_Line_block/Subsystem
  FAULT_findingoutliers_2 : F_Line_block/Subsystem
  newupdateneeded : Logic  AllPortsSameDT=off  OutDataTypeStr=boolean
  FAULT_newupdateneeded : F_Line_block/Subsystem
  FAULT_newupdateneeded_2 : F_Line_block/Subsystem
  nicemeasurementor newupdateneeded : Logic  Operator=OR  AllPortsSameDT=off  OutDataTypeStr=boolean
  FAULT_nicemeasurementor newupdateneeded : F_Line_block/Subsystem
  FAULT_nicemeasurementor newupdateneeded_2 : F_Line_block/Subsystem
  outlierJump : simulink/Logic and Bit Operations/Compare To Constant  relop=<=  const=Estimator.alt.deltaSonarToCurrentMax  OutDataTypeStr=boolean
  FAULT_outlierJump : F_Line_block/Subsystem
  pressureFilter_IIR : DiscreteFilter  Numerator=Estimator.alt.filterPrsNum  Denominator=Estimator.alt.filterPrsDen
  FAULT_pressureFilter_IIR : F_Line_block/Subsystem
  soonarFilter_IIR : DiscreteFilter  Numerator=Estimator.alt.filterSonarNum  Denominator=Estimator.alt.filterSonarDen
  FAULT_soonarFilter_IIR : F_Line_block/Subsystem
  enableKFmeasupdate_flagout : Outport
  FAULT_enableKFmeasupdate_flagout : F_Line_block/Subsystem
  wires:
  Add1/1 -> FAULT_Absestdiff1/1
  FAULT_Absestdiff1/1 -> Absestdiff1/1
  nicemeasurementor newupdateneeded/1 -> FAULT_enableKFmeasupdate_flagout/1
  FAULT_enableKFmeasupdate_flagout/1 -> enableKFmeasupdate_flagout/1
  findingoutliers/1 -> FAULT_nicemeasurementor newupdateneeded/1
  FAULT_nicemeasurementor newupdateneeded/1 -> nicemeasurementor newupdateneeded/1
  check for min altitude/1 -> FAULT_findingoutliers_2/1
  FAULT_findingoutliers_2/1 -> findingoutliers/2
  outlierJump/1 -> FAULT_findingoutliers/1
  FAULT_findingoutliers/1 -> findingoutliers/1
  SaturationSonar/1 -> FAULT_Add/1
  FAULT_Add/1 -> Add/1
  Absestdiff/1 -> FAULT_outlierJump/1
  FAULT_outlierJump/1 -> outlierJump/1
  Add/1 -> FAULT_Absestdiff/1
  FAULT_Absestdiff/1 -> Absestdiff/1
  newupdateneeded/1 -> FAULT_nicemeasurementor newupdateneeded_2/1
  FAULT_nicemeasurementor newupdateneeded_2/1 -> nicemeasurementor newupdateneeded/2
  Absestdiff2/1 -> FAULT_currentStateVeryOffsonarflt/1
  FAULT_currentStateVeryOffsonarflt/1 -> currentStateVeryOffsonarflt/1
  altSonar_datin/1 -> FAULT_SaturationSonar/1, FAULT_soonarFilter_IIR/1, check for min altitude/1
  currentEstimateVeryOffFromPressure/1 -> FAULT_newupdateneeded/1
  FAULT_newupdateneeded/1 -> newupdateneeded/1
  Z_estimin/1 -> FAULT_Add1/1, Add2/1, Add/2
  Add2/1 -> FAULT_Absestdiff2/1
  FAULT_Absestdiff2/1 -> Absestdiff2/1
  currentStateVeryOffsonarflt/1 -> FAULT_newupdateneeded_2/1
  FAULT_newupdateneeded_2/1 -> newupdateneeded/2
  pressureFilter_IIR/1 -> FAULT_Add1_2/1
  FAULT_Add1_2/1 -> Add1/2
  altPrs_datin/1 -> FAULT_pressureFilter_IIR/1
  FAULT_pressureFilter_IIR/1 -> pressureFilter_IIR/1
  soonarFilter_IIR/1 -> FAULT_Add2_2/1
  FAULT_Add2_2/1 -> Add2/2
  Absestdiff1/1 -> FAULT_currentEstimateVeryOffFromPressure/1
  FAULT_currentEstimateVeryOffFromPressure/1 -> currentEstimateVeryOffFromPressure/1

== system FCS/State Estimator/EstimatorXYPosition/EstimatorVelocity ==
  opticalFlow_datin : Inport
  Z_estimin : Inport  Port=2  SampleTime=Ts
  sensorIMU_datin : Inport  Port=3
  orient_estimin : Inport  Port=4
  AccelerationHandling : Subsystem
  DataHandling : Subsystem
  Delay : Delay  DelayLength=1  InitialCondition=0
  FAULT_Delay : F_Line_block/Subsystem
  KalmanFilter_dxdy : ctrlSharedLib/Kalman Filter  TimeDomain=Discrete-Time  UseCurrentEstimator=on  ModelSource=Individual A, B, C, D matrices  ModelSourceVariable=ss(0.95,1,1,0,1)  A=eye(2)  B=Ts*eye(2)  C=eye(2)  D=0  NumberOfStates=1  NumberOfInputs=1  NumberOfOutputs=1  InitialEstimateSource=Dialog  X0=0  P0=10  UseK=off  UseGH=on  NumberOfProcessNoiseInputs=1  G=Estimator.pos.kfVelo.G  TimeInvariantG=on  H=Estimator.pos.kfVelo.H  TimeInvariantH=on  Q=Estimator.pos.kfVelo.Q  TimeInvariantQ=on  R=Estimator.pos.kfVelo.R  TimeInvariantR=on  N=Estimator.pos.kfVelo.N  TimeInvariantN=on  AddInputPort=on  AddEnablePort=on  OutputEstimatedY=off  OutputP=off  Ts=-1
      settings: SourceProductBaseCode=CT
  FAULT_KalmanFilter_dxdy : F_Line_block/Subsystem
  FAULT_KalmanFilter_dxdy_2 : F_Line_block/Subsystem
  FAULT_KalmanFilter_dxdy_3 : F_Line_block/Subsystem
  Select dxy : Selector  InputPortWidth=3  IndexOptions=Index vector (dialog)  Indices=[1 2]  OutputSizes=1
  FAULT_Select dxy : F_Line_block/Subsystem
  opticalFlowToVelocity_gain : Gain  Gain=Estimator.pos.opticalFlowToVelocityGain
  FAULT_opticalFlowToVelocity_gain : F_Line_block/Subsystem
  dxy_estimout : Outport
  FAULT_dxy_estimout : F_Line_block/Subsystem
  wires:
  Delay/1 -> DataHandling/5(dxyOF_datin)
  Z_estimin/1 -> DataHandling/1(Z_estimin), AccelerationHandling/4(Z_estimin)
  KalmanFilter_dxdy/1 -> FAULT_dxy_estimout/1, FAULT_Delay/1
  ?FAULT_Demux1/1 -> ?Demux1/1
  ?FAULT_IIRgyroz/1 -> ?IIRgyroz/1
  FAULT_dxy_estimout/1 -> dxy_estimout/1
  FAULT_Delay/1 -> Delay/1
  opticalFlowToVelocity_gain/1 -> FAULT_Select dxy/1
  FAULT_Select dxy/1 -> Select dxy/1
  opticalFlow_datin/1 -> FAULT_opticalFlowToVelocity_gain/1
  FAULT_opticalFlowToVelocity_gain/1 -> opticalFlowToVelocity_gain/1
  sensorIMU_datin/1 -> AccelerationHandling/2(sensorIMU_datin), DataHandling/3(sensorIMU_datin)
  orient_estimin/1 -> AccelerationHandling/3(orient_estimin), DataHandling/2(orient_estimin)
  Select dxy/1 -> FAULT_KalmanFilter_dxdy_2/1, AccelerationHandling/1(dxy_estimin), DataHandling/4(dxy_estimin)
  AccelerationHandling/1(acceleration_world) -> FAULT_KalmanFilter_dxdy/1
  FAULT_KalmanFilter_dxdy/1 -> KalmanFilter_dxdy/1
  DataHandling/1(enable_flag) -> FAULT_KalmanFilter_dxdy_3/1
  FAULT_KalmanFilter_dxdy_3/1 -> KalmanFilter_dxdy/3

== system FCS/State Estimator/EstimatorXYPosition/EstimatorXYPosition ==
  note: Switching from orientationControl to Position
      | control reset the current world position estimate
      | (happens when using no markers)
  dxy_estimin : Inport
  orient_estimin : Inport  Port=2  SampleTime=Ts
  controlModePosVSOrient_flagin : Inport  Port=3
  dz_estimin : Inport  Port=4
  posVIS_datin : Inport  Port=5
  usePosVIS_flagin : Inport  Port=6
  Delay : Delay  DelayLength=1  InitialCondition=0
  FAULT_Delay : F_Line_block/Subsystem
  KalmanFilter_posxy : ctrlSharedLib/Kalman Filter  TimeDomain=Discrete-Time  UseCurrentEstimator=on  ModelSource=Individual A, B, C, D matrices  ModelSourceVariable=ss(0.95,1,1,0,1)  A=eye(2)  B=Ts*eye(2)  C=eye(2)  D=0  NumberOfStates=1  NumberOfInputs=1  NumberOfOutputs=1  InitialEstimateSource=Dialog  X0=[.1 0]  P0=10  UseK=off  UseGH=on  NumberOfProcessNoiseInputs=1  G=Estimator.pos.kfPos.G  TimeInvariantG=on  H=Estimator.pos.kfPos.H  TimeInvariantH=on  Q=Estimator.pos.kfPos.Q  TimeInvariantQ=on  R=Estimator.pos.kfPos.R  TimeInvariantR=on  N=Estimator.pos.kfPos.N  TimeInvariantN=on  AddInputPort=on  AddEnablePort=on  OutputEstimatedY=off  OutputP=off  Ts=-1
      settings: SourceProductBaseCode=CT
  FAULT_KalmanFilter_posxy : F_Line_block/Subsystem
  FAULT_KalmanFilter_posxy_2 : F_Line_block/Subsystem
  FAULT_KalmanFilter_posxy_3 : F_Line_block/Subsystem
  Math Function : Math  Operator=transpose  SaturateOnIntegerOverflow=on
  FAULT_Math Function : F_Line_block/Subsystem
  Mux2 : Mux  Inputs=2
  FAULT_Mux2 : F_Line_block/Subsystem
  FAULT_Mux2_2 : F_Line_block/Subsystem
  OutlierHandling : Subsystem
  Product : Product  Multiplication=Matrix(*)
  FAULT_Product : F_Line_block/Subsystem
  FAULT_Product_2 : F_Line_block/Subsystem
  Rotation Angles to Direction Cosine Matrix : sharedtransform/Rotation Angles to Direction Cosine Matrix  rotationOrder=ZYX  aMode=aMode
      settings: SourceProductBaseCode=AE
  FAULT_Rotation Angles to Direction Cosine Matrix : F_Line_block/Subsystem
  SelectXY : Selector  InputPortWidth=4  IndexOptions=Index vector (dialog)  Indices=[1 2]  OutputSizes=1
  FAULT_SelectXY : F_Line_block/Subsystem
  SelectdXY : Selector  InputPortWidth=3  IndexOptions=Index vector (dialog)  Indices=[1 2]  OutputSizes=1
  FAULT_SelectdXY : F_Line_block/Subsystem
  SimplyIntegrateVelocity : DiscreteIntegrator  ExternalReset=rising  SampleTime=Ts  ICPrevOutput=DiscIntNeverNeededParam  ICPrevScaledInput=DiscIntNeverNeededParam
  FAULT_SimplyIntegrateVelocity : F_Line_block/Subsystem
  FAULT_SimplyIntegrateVelocity_2 : F_Line_block/Subsystem
  UseIPPosSwitch : Switch  Criteria=u2 > Threshold
  XY_estimout : Outport
  FAULT_XY_estimout : F_Line_block/Subsystem
  wires:
  Delay/1 -> OutlierHandling/3(pos_estim)
  usePosVIS_flagin/1 -> UseIPPosSwitch/2
  UseIPPosSwitch/1 -> FAULT_XY_estimout/1
  FAULT_XY_estimout/1 -> XY_estimout/1
  controlModePosVSOrient_flagin/1 -> FAULT_SimplyIntegrateVelocity_2/1
  FAULT_SimplyIntegrateVelocity_2/1 -> SimplyIntegrateVelocity/2
  KalmanFilter_posxy/1 -> FAULT_Delay/1, UseIPPosSwitch/1
  FAULT_Delay/1 -> Delay/1
  FAULT_SelectXY/1 -> SelectXY/1
  posVIS_datin/1 -> OutlierHandling/2(posVIS_datin), FAULT_SelectXY/1
  FAULT_Delay/1 -> Delay/1
  FAULT_SelectXY/1 -> SelectXY/1
  Product/1 -> FAULT_SelectdXY/1
  FAULT_SelectdXY/1 -> SelectdXY/1
  Mux2/1 -> FAULT_Product_2/1
  FAULT_Product_2/1 -> Product/2
  dz_estimin/1 -> FAULT_Mux2_2/1
  FAULT_Mux2_2/1 -> Mux2/2
  SimplyIntegrateVelocity/1 -> UseIPPosSwitch/3
  dxy_estimin/1 -> FAULT_Mux2/1
  FAULT_Mux2/1 -> Mux2/1
  orient_estimin/1 -> FAULT_Rotation Angles to Direction Cosine Matrix/1, OutlierHandling/1(orient_estimin)
  FAULT_Rotation Angles to Direction Cosine Matrix/1 -> Rotation Angles to Direction Cosine Matrix/1
  FAULT_SelectXY/1 -> SelectXY/1
  Rotation Angles to Direction Cosine Matrix/1 -> FAULT_Math Function/1
  FAULT_Math Function/1 -> Math Function/1
  SelectXY/1 -> FAULT_KalmanFilter_posxy_2/1
  FAULT_KalmanFilter_posxy_2/1 -> KalmanFilter_posxy/2
  OutlierHandling/1(enable_flag) -> FAULT_KalmanFilter_posxy_3/1
  FAULT_KalmanFilter_posxy_3/1 -> KalmanFilter_posxy/3
  SelectdXY/1 -> FAULT_SimplyIntegrateVelocity/1, FAULT_KalmanFilter_posxy/1
  FAULT_SimplyIntegrateVelocity/1 -> SimplyIntegrateVelocity/1
  FAULT_KalmanFilter_posxy/1 -> KalmanFilter_posxy/1
  Math Function/1 -> FAULT_Product/1
  FAULT_Product/1 -> Product/1

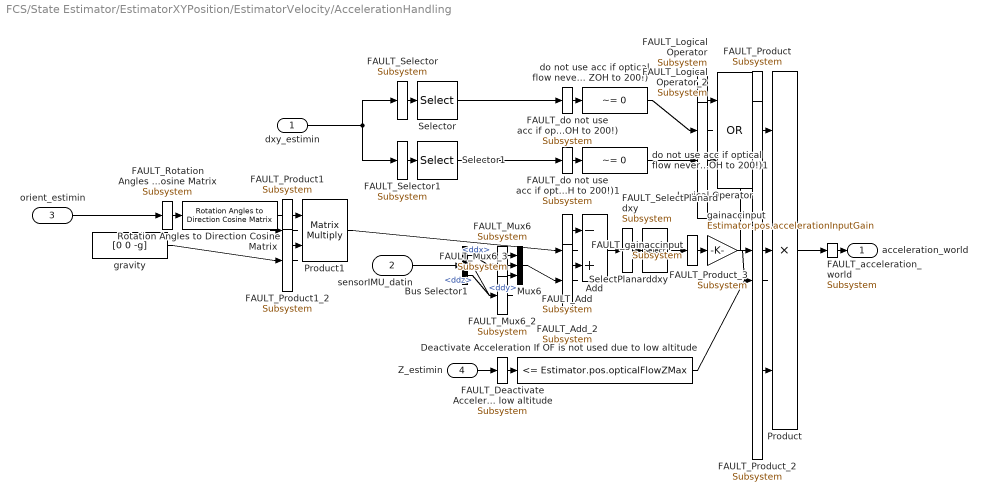
== system FCS/State Estimator/EstimatorXYPosition/EstimatorVelocity/AccelerationHandling ==
  dxy_estimin : Inport
  sensorIMU_datin : Inport  Port=2
  orient_estimin : Inport  Port=3
  Z_estimin : Inport  Port=4
  Add : Sum  Inputs=-+
  FAULT_Add : F_Line_block/Subsystem
  FAULT_Add_2 : F_Line_block/Subsystem
  Bus Selector1 : BusSelector  OutputSignals=ddx,ddy,ddz
  Deactivate Acceleration If OF is not used due to low altitude : simulink/Logic and Bit Operations/Compare To Constant  relop=<=  const=Estimator.pos.opticalFlowZMax  OutDataTypeStr=boolean
  FAULT_Deactivate Acceleration If OF is not used due to low altitude : F_Line_block/Subsystem
  Logical Operator : Logic  Operator=OR  AllPortsSameDT=off  OutDataTypeStr=boolean
  FAULT_Logical Operator : F_Line_block/Subsystem
  FAULT_Logical Operator_2 : F_Line_block/Subsystem
  Mux6 : Mux  Inputs=3
  FAULT_Mux6 : F_Line_block/Subsystem
  FAULT_Mux6_2 : F_Line_block/Subsystem
  FAULT_Mux6_3 : F_Line_block/Subsystem
  Product : Product  Inputs=3
  FAULT_Product : F_Line_block/Subsystem
  FAULT_Product_2 : F_Line_block/Subsystem
  FAULT_Product_3 : F_Line_block/Subsystem
  Product1 : Product  Multiplication=Matrix(*)
  FAULT_Product1 : F_Line_block/Subsystem
  FAULT_Product1_2 : F_Line_block/Subsystem
  Rotation Angles to Direction Cosine Matrix : sharedtransform/Rotation Angles to Direction Cosine Matrix  rotationOrder=ZYX  aMode=aMode
      settings: SourceProductBaseCode=AE
  FAULT_Rotation Angles to Direction Cosine Matrix : F_Line_block/Subsystem
  SelectPlanarddxy : Selector  InputPortWidth=3  IndexOptions=Index vector (dialog)  Indices=[1 2]  OutputSizes=1
  FAULT_SelectPlanarddxy : F_Line_block/Subsystem
  Selector : Selector  InputPortWidth=2  IndexOptions=Index vector (dialog)  Indices=1  OutputSizes=1
  FAULT_Selector : F_Line_block/Subsystem
  Selector1 : Selector  InputPortWidth=2  IndexOptions=Index vector (dialog)  Indices=2  OutputSizes=1
  FAULT_Selector1 : F_Line_block/Subsystem
  do not use acc if optical flow never available (Note OF@60Hz but ZOH to 200!) : simulink/Logic and Bit Operations/Compare To Constant  relop=~=  const=0  OutDataTypeStr=boolean
  FAULT_do not use acc if optical flow never available (Note OF@60Hz but ZOH to 200!) : F_Line_block/Subsystem
  do not use acc if optical flow never available (Note OF@60Hz but ZOH to 200!)1 : simulink/Logic and Bit Operations/Compare To Constant  relop=~=  const=0  OutDataTypeStr=boolean
  FAULT_do not use acc if optical flow never available (Note OF@60Hz but ZOH to 200!)1 : F_Line_block/Subsystem
  gainaccinput : Gain  Gain=Estimator.pos.accelerationInputGain  OutDataTypeStr=single
  FAULT_gainaccinput : F_Line_block/Subsystem
  gravity : Constant  Value=[0 0 -g]
  acceleration_world : Outport  OutDataTypeStr=single
  FAULT_acceleration_world : F_Line_block/Subsystem
  wires:
  do not use acc if optical flow never available (Note OF@60Hz but ZOH to 200!)1/1 -> FAULT_Logical Operator_2/1
  FAULT_Logical Operator_2/1 -> Logical Operator/2
  do not use acc if optical flow never available (Note OF@60Hz but ZOH to 200!)/1 -> FAULT_Logical Operator/1
  FAULT_Logical Operator/1 -> Logical Operator/1
  Logical Operator/1 -> FAULT_Product/1
  FAULT_Product/1 -> Product/1
  Selector1/1 -> FAULT_do not use acc if optical flow never available (Note OF@60Hz but ZOH to 200!)1/1
  FAULT_do not use acc if optical flow never available (Note OF@60Hz but ZOH to 200!)1/1 -> do not use acc if optical flow never available (Note OF@60Hz but ZOH to 200!)1/1
  Selector/1 -> FAULT_do not use acc if optical flow never available (Note OF@60Hz but ZOH to 200!)/1
  FAULT_do not use acc if optical flow never available (Note OF@60Hz but ZOH to 200!)/1 -> do not use acc if optical flow never available (Note OF@60Hz but ZOH to 200!)/1
  dxy_estimin/1 -> FAULT_Selector1/1, FAULT_Selector/1
  FAULT_Selector1/1 -> Selector1/1
  FAULT_Selector/1 -> Selector/1
  Product/1 -> FAULT_acceleration_world/1
  FAULT_acceleration_world/1 -> acceleration_world/1
  Deactivate Acceleration If OF is not used due to low altitude/1 -> FAULT_Product_3/1
  FAULT_Product_3/1 -> Product/3
  Z_estimin/1 -> FAULT_Deactivate Acceleration If OF is not used due to low altitude/1
  FAULT_Deactivate Acceleration If OF is not used due to low altitude/1 -> Deactivate Acceleration If OF is not used due to low altitude/1
  Add/1 -> FAULT_SelectPlanarddxy/1
  FAULT_SelectPlanarddxy/1 -> SelectPlanarddxy/1
  Product1/1 -> FAULT_Add/1
  FAULT_Add/1 -> Add/1
  gravity/1 -> FAULT_Product1_2/1
  FAULT_Product1_2/1 -> Product1/2
  gainaccinput/1 -> FAULT_Product_2/1
  FAULT_Product_2/1 -> Product/2
  SelectPlanarddxy/1 -> FAULT_gainaccinput/1
  FAULT_gainaccinput/1 -> gainaccinput/1
  Bus Selector1/3 -> FAULT_Mux6_3/1  "<ddz>"
  FAULT_Mux6_3/1 -> Mux6/3
  Bus Selector1/1 -> FAULT_Mux6/1  "<ddx>"
  FAULT_Mux6/1 -> Mux6/1
  sensorIMU_datin/1 -> Bus Selector1/1
  Mux6/1 -> FAULT_Add_2/1
  FAULT_Add_2/1 -> Add/2
  Bus Selector1/2 -> FAULT_Mux6_2/1  "<ddy>"
  FAULT_Mux6_2/1 -> Mux6/2
  orient_estimin/1 -> FAULT_Rotation Angles to Direction Cosine Matrix/1
  FAULT_Rotation Angles to Direction Cosine Matrix/1 -> Rotation Angles to Direction Cosine Matrix/1
  Rotation Angles to Direction Cosine Matrix/1 -> FAULT_Product1/1
  FAULT_Product1/1 -> Product1/1
